simulink model "Zad_1_szybkozmienny"  (R2018a)
settings: Solver=FixedStepAuto  StartTime=0.0  StopTime=0  MaxStep=0  RelTol=1e-3
libraries: CPOiS_SourcesSinks x4, CPOiS_DataManipulation x2, CPOiS_General x1
settings Model: Creator=rafal  LastModifiedBy=rafal

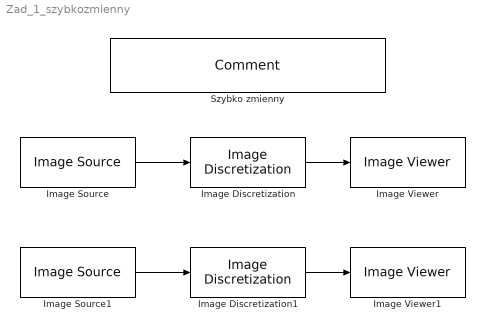
== system Zad_1_szybkozmienny ==
  Image Discretization : CPOiS_DataManipulation/Image Discretization  factor=2
      settings: SourceProductName=CPOiS - Digital image and signal processing
  Image Discretization1 : CPOiS_DataManipulation/Image Discretization  factor=4
      settings: SourceProductName=CPOiS - Digital image and signal processing
  Image Source : CPOiS_SourcesSinks/Image Source  FileSelection=gull.png
      settings: SourceProductName=CPOiS - Digital image and signal processing
  Image Source1 : CPOiS_SourcesSinks/Image Source  FileSelection=gull.png
      settings: SourceProductName=CPOiS - Digital image and signal processing
  Image Viewer : CPOiS_SourcesSinks/Image Viewer
      settings: SourceProductName=CPOiS - Digital image and signal processing
  Image Viewer1 : CPOiS_SourcesSinks/Image Viewer
      settings: SourceProductName=CPOiS - Digital image and signal processing
  Szybko zmienny : CPOiS_General/Comment
      settings: SourceProductName=CPOiS - Digital image and signal processing
  wires:
  Image Source/1 -> Image Discretization/1
  Image Discretization/1 -> Image Viewer/1
  Image Source1/1 -> Image Discretization1/1
  Image Discretization1/1 -> Image Viewer1/1
